simulink model "lab2_2"  (R2021a)
settings: Solver=VariableStepAuto  StartTime=0.0  StopTime=10.0  RelTol=10e-10  AbsTol=10e-10
values from neighbouring files (symbols this model uses):
  g = 9.81    [lab2.m]
  km = 0.1    [lab2.m]
  La = 0.05    [lab2.m]
  M = 0.1    [lab2.m]
  Ra = 3    [lab2.m]
  ubar = 3*ybar*sqrt(g)    [lab2.m]
  ybar = 0.1    [lab2.m]
libraries: cstblocks x1
settings Model: Creator=markalex  LastModifiedBy=markalex

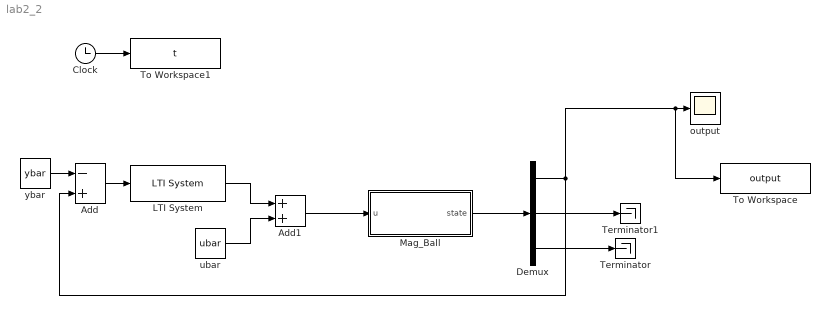
== system lab2_2 ==
  Add : Sum  Inputs=-+
  Add1 : Sum
  Clock : Clock
  Demux : Demux  Outputs=3
  LTI System : cstblocks/LTI System  sys=CONTROLLER  IC=[]
  Mag_Ball : Subsystem
  Terminator : Terminator
  Terminator1 : Terminator
  To Workspace : ToWorkspace  VariableName=output  SampleTime=1e-3
  To Workspace1 : ToWorkspace  VariableName=t  SampleTime=1e-3
  output : Scope
  ubar : Constant  Value=ubar
  ybar : Constant  Value=ybar
  wires:
  Mag_Ball/1(state) -> Demux/1
  Demux/1 -> Add/2, To Workspace/1, output/1
  Demux/2 -> Terminator1/1
  Demux/3 -> Terminator/1
  ybar/1 -> Add/1
  Add/1 -> LTI System/1
  LTI System/1 -> Add1/1
  Add1/1 -> Mag_Ball/1(u)
  ubar/1 -> Add1/2
  Clock/1 -> To Workspace1/1

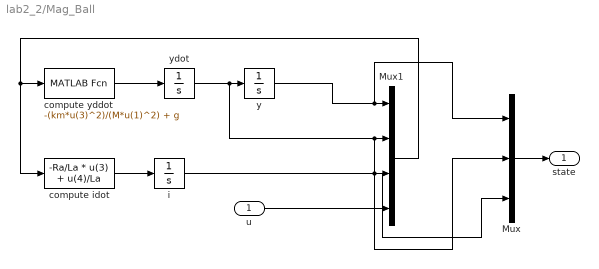
== system lab2_2/Mag_Ball ==
  u : Inport
  Mux : Mux  Inputs=3
  Mux1 : Mux
  compute idot : MATLABFcn  MATLABFcn=-Ra/La * u(3) + u(4)/La
  compute yddot : MATLABFcn  MATLABFcn=-(km*u(3)^2)/(M*u(1)^2) + g
  i : Integrator
  y : Integrator  InitialCondition=0.15
  ydot : Integrator
  state : Outport
  wires:
  u/1 -> Mux1/4
  compute idot/1 -> i/1
  i/1 -> Mux/3, Mux1/3
  y/1 -> Mux/1, Mux1/1
  ydot/1 -> Mux/2, Mux1/2, y/1
  compute yddot/1 -> ydot/1
  Mux/1 -> state/1
  Mux1/1 -> compute idot/1, compute yddot/1
